simulink model "BLDCmotor_FOC_R2017b_fixdt"  (R2025a)
settings: Solver=FixedStepDiscrete  StartTime=0  StopTime=0.5  FixedStep=Ts  MaxStep=1e-6  RelTol=1e-6  AbsTol=1e-6  EnableMultiTasking=on
PreLoadFcn:
  | addpath(pwd);
  | addpath(genpath('01_Libraries'));
  | addpath(genpath('02_Figures'));
  | addpath(genpath('03_CreateParamTable'));
InitFcn:
  | init_model;
values from neighbouring files (symbols this model uses):
  a_cpr = 65535    [init_model.m]
  a_elecAngle = 60    [init_model.m]
  a_elecoffset = a_elecPeriod/12    (= 30)    [init_model.m]
  a_elecPeriod = 360    [init_model.m]
  a_fcpr = 1/65535    (= 1.52590218967e-05)    [init_model.m]
  a_mechoffset = a_elecoffset/n_polePairs    (= 5)    [init_model.m]
  a_phaAdvMax = 25    [init_model.m]
  b_angleMeasEna = 1    [init_model.m]
  b_cruiseCtrlEna = 0    [init_model.m]
  b_diagEna = 0    [init_model.m]
  b_fieldWeakEna = 0    [init_model.m]
  cf_currFilt = 0.692    [init_model.m]
  cf_idKi = Ki / (f_ctrl)    (= 0.00409061543436)    [init_model.m]
  cf_idKp = Kp    (= 0.0523598775598)    [init_model.m]
  cf_iqKi = Ki / (f_ctrl)    (= 0.00409061543436)    [init_model.m]
  cf_iqKiLimProt = 60 / (f_ctrl)    (= 0.00375)    [init_model.m]
  cf_iqKp = Kp    (= 0.0523598775598)    [init_model.m]
  cf_KbLimProt = Simulink.Parameter    [init_model.m]
  cf_nKi = 20.4 / (f_ctrl)    (= 0.001275)    [init_model.m]
  cf_nKiLimProt = 20 / (f_ctrl)    (= 0.00125)    [init_model.m]
  cf_nKp = 1.18    [init_model.m]
  cf_speedCoef = round(f_ctrl * a_mechAngle * (pi/180) * (30/pi))    [init_model.m]
  CTRL_FOC = 2    [init_model.m]
  CTRL_SIN = 1    [init_model.m]
  dV_openRate = 1000 / (f_ctrl)    (= 0.0625)    [init_model.m]
  dz_cntTrnsDetHi = 40    [init_model.m]
  dz_cntTrnsDetLo = 20    [init_model.m]
  ff_gain = ((r_motn / i_sca) * ((GD32_Vd_max_margin) / v_bus))    (= 0.338958333333)    [init_model.m]
  GD32_Vd_max_margin = GD32_Vd_max - V_margin    (= 1627)    [init_model.m]
  GD32_Vq_max_M1 = sqrt(GD32_Vd_max_margin^2 - GD32_Vq_max_XA.^2)    [init_model.m]
  i_max = i_max * i_sca    (= 500)    [init_model.m]
  id_fieldWeakMax = 5 * i_sca    (= 250)    [init_model.m]
  iq_maxSca_M1 = sqrt(1 - iq_maxSca_XA.^2)    [init_model.m]
  mcu_model = GD32F103    (= 1)    [init_model.m]
  n_commAcvLo = 15    [init_model.m]
  n_commDeacvHi = 30    [init_model.m]
  n_cruiseMotTgt = 0    [init_model.m]
  n_fieldWeakAuthHi = 300    [init_model.m]
  n_fieldWeakAuthLo = 100    [init_model.m]
  n_max = 1950    [init_model.m]
  n_polePairs = 6    [init_model.m]
  n_stdStillDet = 3    [init_model.m]
  OPEN_MODE = 0    [init_model.m]
  r_cos_M1 = cos((a_elecAngle_XA + a_elecPeriod/12)*(pi/180))    [init_model.m]
  r_errInpTgtThres = 600    [init_model.m]
  r_fieldWeakHi = 1000    [init_model.m]
  r_fieldWeakLo = 750    [init_model.m]
  r_motn = r_mot/2    (= 0.25)    [init_model.m]
  r_sin3PhaA_M1 = sin3Arm + A*r_sinPhaA_M1    [init_model.m]
  r_sin3PhaB_M1 = sin3Arm + A*r_sinPhaB_M1    [init_model.m]
  r_sin3PhaC_M1 = sin3Arm + A*r_sinPhaC_M1    [init_model.m]
  r_sin_M1 = sin((a_elecAngle_XA + a_elecPeriod/12)*(pi/180))    [init_model.m]
  SPD_MODE = 2    [init_model.m]
  STM32_Vd_max_margin = STM32_Vd_max - V_margin    (= 940)    [init_model.m]
  STM32_Vq_max_M1 = sqrt(STM32_Vd_max_margin^2 - STM32_Vq_max_XA.^2)    [init_model.m]
  t_errDequal = 1.80 * f_ctrl    (= 28800)    [init_model.m]
  t_errQual = 0.24 * f_ctrl    (= 3840)    [init_model.m]
  tgt_scale = 2047    [init_model.m]
  TRQ_MODE = 3    [init_model.m]
  Ts = 5e-6    (= 5e-06)    [init_model.m]
  Ts_ctrl = 6e-5    (= 6e-05)    [init_model.m]
  v_bus = 24    [init_model.m]
  vec_hallToPos = [0 2 0 1 4 3 5 0]    [init_model.m]
  VLT_MODE = 1    [init_model.m]
  z_commutMap_M1 = [-1 -1  0  1  1  0 ... (first row only)    [init_model.m]
  z_ctrlModReq = TRQ_MODE    (= 3)    [init_model.m]
  z_ctrlTypSel = CTRL_FOC    (= 2)    [init_model.m]
  z_maxCntRst = 2000    [init_model.m]
  z_selPhaCurMeasABC = 2    [init_model.m]
undefined symbols (not defined in the file or in its folder): BLDCmotor_FOC_R2017b_fixdt, DiscIntNeverNeededParam, DWORK0, DWORK1, DWORK2, DWORK3, powergui, spspowerguiLib
libraries: BLDC_controller_Lib x18, simulink x13, prociolib x6, eePwmGenerator x6, eePwmGeneratorMultilevel x3, mcbpositiondecoderlib x2, slpidlib x2, spsControlledVoltageSourceLib x1, spsMultimeterLib x1, spsPermanentMagnetSynchronousMachineLib x1, spsUniversalBridgeLib x1, spsVoltageMeasurementLib x1
(part 1 of 6)
Description:
  | This model implements FOC controller for a BLDC motor.
  | The controller is capable for embedded code generation.
  | 
  | Copyright © 2019-2020 Emanuel FERU
settings Model: ExtModeAutoUpdateStatusClock=off  TunableVars=Vd_max,Vq_max_M1,Vq_max_XA,a_phaAdvMax,b_angleMeasEna,b_cruiseCtrlEna,b_diagEna,b_fieldWeakEna,cf_currFilt,cf_idKi,cf_idKp,cf_iqKi,cf_iqKiLimProt,cf_iqKp,cf_nKi,cf_nKiLimProt,cf_nKp,cf_speedCoef,dV_openRate,dz_cntTrnsDetHi,dz_cntTrnsDetLo,i_max,id_fieldWeakMax,n_commAcvLo,n_commDeacvHi,n_cruiseMotTgt,n_fieldWeakAuthHi,n_fieldWeakAuthLo,n_max,n_polePairs,n_stdStillDet,r_errInpTgtThres,r_fieldWeakHi,r_fieldWeakLo,t_errDequal,t_errQual,z_ctrlTypSel,z_maxCntRst,z_selPhaCurMeasABC,sca_factor,ff_gain,a_cpr,a_fcpr  TunableVarsStorageClass=Auto,Auto,Auto,Auto,Auto,Auto,Auto,Auto,Auto,Auto,Auto,Auto,Auto,Auto,Auto,Auto,Auto,Auto,Auto,Auto,Auto,Auto,Auto,Auto,Auto,Auto,Auto,Auto,Auto,Auto,Auto,Auto,Auto,Auto,Auto,Auto,Auto,Auto,Auto,ExportedGlobal,Auto,Auto,Auto  TunableVarsTypeQualifier=,,,,,,,,,,,,,,,,,,,,,,,,,,,,,,,,,,,,,,,,,,  Creator=MathWorks  LastModifiedBy=ernes
settings SolverCC: AutoScaleAbsTol=off  AlgebraicLoopSolver=TrustRegion  AutoInsertRateTranBlk=on
settings DataIOCC: LimitDataPoints=on  SaveFormat=Array  SignalLoggingName=sigsOut
settings OptimizationCC: DefaultParameterBehavior=Inlined  UseDivisionForNetSlopeComputation=on  UseFloatMulNetSlope=on  DefaultUnderspecifiedDataType=single  UseSpecifiedMinMax=on  PassReuseOutputArgsAs=Individual arguments  ExpressionDepthLimit=2147483647.0  ZeroExternalMemoryAtStartup=off  ZeroInternalMemoryAtStartup=off  NoFixptDivByZeroProtection=on  EfficientFloat2IntCast=on  LifeSpan=1  MaxStackSize=64  SimCompilerOptimization=on  OptimizeBlockOrder=speed  DifferentSizesBufferReuse=on  EfficientTunableParamExpr=on
settings DebuggingCC: SignalRangeChecking=warning  ReadBeforeWriteMsg=DisableAll  WriteAfterWriteMsg=DisableAll  WriteAfterReadMsg=DisableAll  InheritedTsInSrcMsg=none  MultiTaskDSMMsg=none  MultiTaskCondExecSysMsg=none  ParamPrecisionLossAbsoluteDiffThreshold=10e-05  ParamPrecisionLossRelativeDiffThreshold=10e-05  ParameterTunabilityLossMsg=error  UnconnectedInputMsg=warning  UnconnectedOutputMsg=warning  UnconnectedLineMsg=warning  StateNameClashWarn=warning  SFUnexpectedBacktrackingDiag=warning  SFNoUnconditionalDefaultTransitionDiag=warning  SFExecutionAtInitializationDiag=none  ArithmeticOperatorsInVariantConditions=warning
settings HardwareCC: ProdBitPerPointer=32.0  ProdBitPerSizeT=32.0  ProdBitPerPtrDiffT=32.0  ProdLargestAtomicInteger=Long  ProdLargestAtomicFloat=Double  ProdWordSize=32.0  ProdLongLongMode=on  ProdHWDeviceType=ARM Compatible->ARM Cortex-M  TargetBitPerPointer=64.0  TargetBitPerSizeT=64.0  TargetBitPerPtrDiffT=64.0  TargetLongLongMode=on  TargetIntDivRoundTo=Zero  TargetEndianess=LittleEndian  TargetWordSize=64.0  TargetHWDeviceType=MATLAB Host  ProdEqTarget=off
settings ModelReferenceCC: UpdateModelReferenceTargets=IfOutOfDate  EnableRefExpFcnMdlSchedulingChecks=on  PropagateSignalLabelsOutOfModel=off
settings SFSimCC: SFSimEcho=off  SimUseLocalCustomCode=off  MATLABDynamicMemAlloc=off  CustomCodeUndefinedFunction=UseInterfaceOnly  SimGPUCompilerFlags="-allow-unsupported-compiler -ccbin \"C:\\Program Files (x86)\\Microsoft Visual Studio\\2022\\BuildTools\\VC\\Tools\\MSVC\\14.29.30133\\bin\\Hostx64\\x64\""
settings RTWCC: SystemTargetFile=ert.tlc  GenCodeOnly=on  TemplateMakefile=ert_default_tmf  GenerateReport=on  RetainRTWFile=on  RTWUseLocalCustomCode=off  Toolchain=GNU Tools for ARM Embedded Processors  BuildConfiguration=Faster Runs  IncludeHyperlinkInReport=on  LaunchReport=on  GenerateTraceInfo=on  GenerateTraceReport=on  GenerateTraceReportSl=on  GenerateTraceReportSf=on  GenerateTraceReportEml=on  GenerateWebview=on  GenerateCodeMetricsReport=on  GenerateCodeReplacementReport=on  GPUComputeCapability=3.5  Description=Embedded Coder
settings CodeAppCC: ForceParamTrailComments=on  IgnoreCustomStorageClasses=off  OperatorAnnotations=on  SimulinkDataObjDesc=on  SFDataObjDesc=on  CustomSymbolStrGlobalVar=rt$N$M  CustomSymbolStrType=$N$M  CustomSymbolStrFcn=$N$M$F  CustomSymbolStrMacro=$N$M  SignalNamingFcn=init_model.m  InsertBlockDesc=on
settings ERTTargetCC: ExtModeTransport=3.0  ExtModeStaticAllocSize=2048.0  InlinedParameterPlacement=Hierarchical  MultiInstanceErrorCode=None  RootIOFormat=Part of model data structure  ERTCustomFileTemplate=example_file_process.tlc  ERTFilePackagingFormat=CompactWithDataFile  PreserveStaticInFcnDecls=off  DynamicArrayContainerType=coder::array  TargetLangStandard=C99 (ISO)  IncludeMdlTerminateFcn=off  CombineSignalStateStructs=on  SuppressErrorStatus=on  CodeInterfacePackaging=Reusable function  PurelyIntegerCode=on  SupportNonFinite=off  SupportComplex=off
settings ConfigComp: CovScope=ReferencedModels  CovMetricSettings=dw  CovSaveCumulativeToWorkspaceVar=on  CovSaveSingleToWorkspaceVar=on  CovExternalEMLEnable=off  CovSFcnEnable=off
settings SimscapeCC: SimscapeNormalizeSystem=off

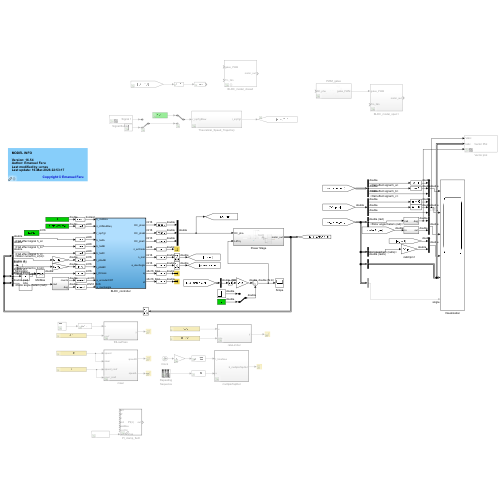
[thumbnail: Simulink's stored preview of the top-level diagram]
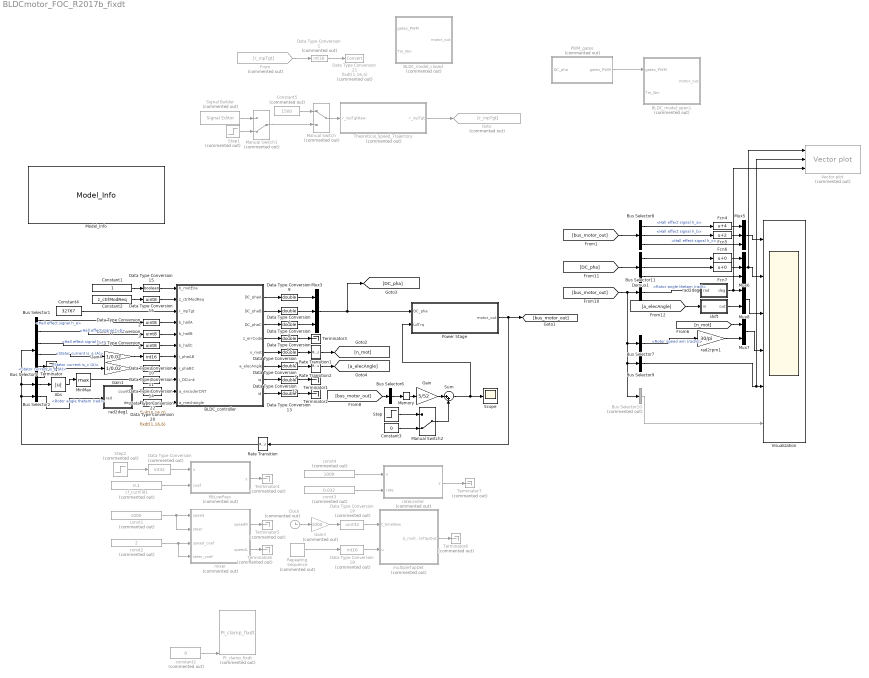
== system BLDCmotor_FOC_R2017b_fixdt ==
  Abs : Abs  SaturateOnIntegerOverflow=off
  BLDC_controller : Subsystem  TreatAsAtomicUnit=on  SystemSampleTime=Ts_ctrl
      settings: RTWFileNameOpts=Use subsystem name  FunctionWithSeparateData=on
  BLDC_model_closed : Subsystem  Commented=on
      mask help: Simulink:masks:GenSFuncDesc_MD
      mask Help: eval('feval(''rtwprivate'',''rtwhelpview'',''rtw_sfcn_block'')');
  BLDC_model_open1 : Subsystem  Commented=on
  Bus Selector1 : BusSelector  OutputSignals=Hall effect signal h_a,Hall effect signal h_b,Hall effect signal h_c,Stator current is_a (A),Stator current is_b (A),Stator current is_c (A)
  Bus Selector10 : BusSelector  Commented=on  OutputSignals=Stator back EMF e_b (V),Stator back EMF e_cV)  OutputAsBus=on
  Bus Selector11 : BusSelector  OutputSignals=Rotor angle thetam (rad)
  Bus Selector2 : BusSelector  OutputSignals=Rotor angle thetam (rad)
  Bus Selector5 : BusSelector  OutputSignals=Electromagnetic torque Te (N*m)  OutputAsBus=on
  Bus Selector6 : BusSelector  OutputSignals=Electromagnetic torque Te (N*m)  OutputAsBus=on
  Bus Selector7 : BusSelector  OutputSignals=Rotor speed wm (rad/s)
  Bus Selector8 : BusSelector  OutputSignals=Hall effect signal h_a,Hall effect signal h_b,Hall effect signal h_c
  Bus Selector9 : BusSelector  OutputSignals=Stator current is_a (A),Stator current is_b (A),Stator current is_c (A),Electromagnetic torque Te (N*m)  OutputAsBus=on
  Clock : Clock  Commented=on
  Constant1 : Constant  OutDataTypeStr=double
  Constant2 : Constant  Value=z_ctrlModReq  OutDataTypeStr=double
  Constant3 : Constant  Value=0  OutDataTypeStr=double
  Constant4 : Constant  Value=32767  OutDataTypeStr=int16
  Constant5 : Constant  Commented=on  Value=1500  OutDataTypeStr=double
  Data Type Conversion : DataTypeConversion  Commented=on  OutDataTypeStr=int32  SaturateOnIntegerOverflow=off  RndMeth=Floor
  Data Type Conversion1 : DataTypeConversion  Commented=on  OutDataTypeStr=int16  SaturateOnIntegerOverflow=off
  Data Type Conversion10 : DataTypeConversion  OutDataTypeStr=int16
  Data Type Conversion11 : DataTypeConversion  OutDataTypeStr=int16
  Data Type Conversion{5..9,12..13,17} (8 alike) : DataTypeConversion  OutDataTypeStr=double  SaturateOnIntegerOverflow=off
  Data Type Conversion14 : DataTypeConversion  OutDataTypeStr=int16
  Data Type Conversion15 : DataTypeConversion  OutDataTypeStr=boolean  SaturateOnIntegerOverflow=off
  Data Type Conversion{2..4,16} (4 alike) : DataTypeConversion  OutDataTypeStr=uint8  SaturateOnIntegerOverflow=off
  Data Type Conversion18 : DataTypeConversion  Commented=on  OutDataTypeStr=int16  SaturateOnIntegerOverflow=off  RndMeth=Floor
  Data Type Conversion19 : DataTypeConversion  Commented=on  OutDataTypeStr=uint32  SaturateOnIntegerOverflow=off  RndMeth=Floor
  Data Type Conversion20 : DataTypeConversion  OutDataTypeStr=fixdt(1,16,6)  SaturateOnIntegerOverflow=off  RndMeth=Floor
  Data Type Conversion21 : DataTypeConversion  Commented=on  OutDataTypeStr=fixdt(1,16,4)  SaturateOnIntegerOverflow=off  RndMeth=Floor
  Data Type Conversion22 : DataTypeConversion  OutDataTypeStr=fixdt(0,16,0)  SaturateOnIntegerOverflow=off  RndMeth=Floor
  Demux1 : Demux  Outputs=3
  Fcn4 : Fcn  Expr=u+4
  Fcn5 : Fcn  Expr=u+2
  Fcn6 : Fcn  Expr=u+0
  Fcn7 : Fcn  Expr=u+0
  From : From  Commented=on  GotoTag=r_inpTgt
  Gain : Gain  Gain=5/52
  Gain1 : Gain  Tag=struct('comment',struct('text','','placement',1),'logdata',struct('maxnumvals',inf,'plotchannels',[],'loggingmode',3,'channels',1),'output',struct('variable','','description','','name','$S_$B','width',1,'address','','max',NaN,'min',NaN,'class','default','type','CONTINUOUS','scaling','','lsb',1,'offset',0,'arb',0,'freeze',1,'unit','','autoscalingmode',1,'lowerheadroom',1,'upperheadroom',1,'headroomunit','bit','keepdatatype',1,'checkmin',0,'checkmax',0,'castoutput',0,'show',0),'gain',struct('variable','','description','','name','$S_$B_gain','width',1,'address','','max',NaN,'min',NaN,'class','default','type','CONTINUOUS','scaling','','lsb',1,'offset',0,'arb',0,'freeze',1,'unit','','keepdatatype',1,'value','1','scalar',0,'tolerance',1),'scalingvalid',0,'date',730486)  Gain=1/0.02  RndMeth=Zero  SaturateOnIntegerOverflow=on  OutDataTypeStr=Inherit: Same as input  ParamDataTypeStr=Inherit: Same as input
  Gain3 : Gain  Tag=struct('comment',struct('text','','placement',1),'logdata',struct('maxnumvals',inf,'plotchannels',[],'loggingmode',3,'channels',1),'output',struct('variable','','description','','name','$S_$B','width',1,'address','','max',NaN,'min',NaN,'class','default','type','CONTINUOUS','scaling','','lsb',1,'offset',0,'arb',0,'freeze',1,'unit','','autoscalingmode',1,'lowerheadroom',1,'upperheadroom',1,'headroomunit','bit','keepdatatype',1,'checkmin',0,'checkmax',0,'castoutput',0,'show',0),'gain',struct('variable','','description','','name','$S_$B_gain','width',1,'address','','max',NaN,'min',NaN,'class','default','type','CONTINUOUS','scaling','','lsb',1,'offset',0,'arb',0,'freeze',1,'unit','','keepdatatype',1,'value','1','scalar',0,'tolerance',1),'scalingvalid',0,'date',730486)  Commented=on  Gain=1000  RndMeth=Zero  SaturateOnIntegerOverflow=on  OutDataTypeStr=Inherit: Same as input  ParamDataTypeStr=Inherit: Same as input
  Gain4 : Gain  Tag=struct('comment',struct('text','','placement',1),'logdata',struct('maxnumvals',inf,'plotchannels',[],'loggingmode',3,'channels',1),'output',struct('variable','','description','','name','$S_$B','width',1,'address','','max',NaN,'min',NaN,'class','default','type','CONTINUOUS','scaling','','lsb',1,'offset',0,'arb',0,'freeze',1,'unit','','autoscalingmode',1,'lowerheadroom',1,'upperheadroom',1,'headroomunit','bit','keepdatatype',1,'checkmin',0,'checkmax',0,'castoutput',0,'show',0),'gain',struct('variable','','description','','name','$S_$B_gain','width',1,'address','','max',NaN,'min',NaN,'class','default','type','CONTINUOUS','scaling','','lsb',1,'offset',0,'arb',0,'freeze',1,'unit','','keepdatatype',1,'value','1','scalar',0,'tolerance',1),'scalingvalid',0,'date',730486)  Gain=1/0.02  RndMeth=Zero  SaturateOnIntegerOverflow=on  OutDataTypeStr=Inherit: Same as input  ParamDataTypeStr=Inherit: Same as input
  Goto : Goto  Commented=on  GotoTag=r_inpTgt
  Manual Switch : ManualSwitch  Commented=on
  Manual Switch1 : ManualSwitch  Commented=on  CurrentSetting=0
  Manual Switch2 : ManualSwitch  CurrentSetting=0
  Memory : Memory
  MinMax : MinMax  Function=max
  Model_Info : BLDC_controller_Lib/Model_Info
  Mux3 : Mux  Inputs=3
  Mux5 : Mux  Inputs=3
  Mux6 : Mux  Inputs=3
  Mux7 : Mux  Inputs=2
  Mux8 : Mux  Inputs=2
  PI_clamp_fixdt : BLDC_controller_Lib/PI_clamp_fixdt  Commented=on  SystemSampleTime=-1  VariantActivationTime=update diagram  EmptyChoice=off  PassThrough=off  PassThroughVariantControl=(default)  EmptyChoiceVariantControl=(default)  AllowFlexibleInterface=on  Latency=0  AutoFrameSizeCalculation=off
  PWM_gates : Subsystem  Commented=on
  Power Stage : Subsystem
  Rate Transition : RateTransition  Integrity=off  Deterministic=off
  Rate Transition1 : RateTransition  Integrity=off  Deterministic=off
  Rate Transition2 : RateTransition
  Repeating Sequence : simulink/Sources/Repeating Sequence  Commented=on  rep_seq_t=[0 0.4 0.8 1.2 1.6 3]  rep_seq_y="[0 900  0  900 0 0]"
  Scope : Scope
      settings: ActiveDisplayYMinimum=-7.8527501814410146  ActiveDisplayYMaximum=12.467804815111347  DataLoggingVariableName=ScopeData2
  Signal Builder : SignalEditorBlockLib/Signal Editor  Commented=on  FileName=SignalBuilder_2.mat  ActiveScenario=Group_1  ActiveSignal=Signal 1  IsBus=off  OutputBusObjectStr=Bus: BusObject  SampleTime=-1  OutputAfterFinalValue=Extrapolation  Unit=inherit  PreserveSignalName=on  ApplySigPropsToAllScenarios=on  ApplySigPropsToAllSignals=off  SignalPropertySource=Dialog parameters
  Step : Step  Time=0.25  Before=-5  After=5  SampleTime=0
  Step1 : Step  Commented=on  Time=0.25  Before=1500  After=-1500
  Step2 : Step  Commented=on  Time=0.25  Before=20000  After=0  OutDataTypeStr=single  SampleTime=0
  Sum : Sum  Inputs=|++
  Terminator{,1..3} (4 alike) : Terminator
      Terminator1 settings: Tag=Controls_Lib  Description=Terminator  CopyFcn=Lib_CopyFcn(gcb);  PreDeleteFcn=Lib_PreDeleteFcn(gcb);
      Terminator2 settings: Tag=Controls_Lib  Description=Terminator  CopyFcn=Lib_CopyFcn(gcb);  PreDeleteFcn=Lib_PreDeleteFcn(gcb);
      Terminator3 settings: Tag=Controls_Lib  Description=Terminator  CopyFcn=Lib_CopyFcn(gcb);  PreDeleteFcn=Lib_PreDeleteFcn(gcb);
  Terminator{4..8} (5 alike) : Terminator  Commented=on
      settings: Tag=Controls_Lib  Description=Terminator  CopyFcn=Lib_CopyFcn(gcb);  PreDeleteFcn=Lib_PreDeleteFcn(gcb);
  Theoretical_Speed_Trajectory : Subsystem  Commented=on
  Vector plot : mcbutilslib/Vector plot  Commented=on  InputSignals=Vabc Iabc Theta  ReferenceFrame=Rotating Reference Frame  axisAlign=Q-axis  thetaUnits=Degrees  angleUnits=Radians  OpenFigAtSimStart=off  debugEnable=0
      settings: LibrarySourceBlock=mcblib/Signal Management/Vector plot
  Visualization : Scope  NumInputPorts=6
      settings: TimeSpan=0.2  ActiveDisplayString=4  ActiveDisplayYMinimum=-21.20436412488284  ActiveDisplayYMaximum=402.88291837277404
  cf_currFilt1 : Constant  Commented=on  Value=0.1  OutDataTypeStr=fixdt(0,16,16)
  const1 : Constant  Commented=on  Value=1000  OutDataTypeStr=fixdt(1,16,4)
  const2 : Constant  Commented=on  Value=2  OutDataTypeStr=fixdt(1,16,14)
  const3 : Constant  Commented=on  Value=0.032  OutDataTypeStr=fixdt(1,16,4)
  const4 : Constant  Commented=on  Value=1000  OutDataTypeStr=int16
  constant2 : Constant  Commented=on  Value=0  OutDataTypeStr=Inherit: Inherit via back propagation
  filtLowPass : Subsystem  Commented=on  TreatAsAtomicUnit=on  SystemSampleTime=Ts_ctrl
      settings: RTWFcnNameOpts=Use subsystem name
  mixer : Subsystem  Commented=on  TreatAsAtomicUnit=on  SystemSampleTime=Ts_ctrl
      settings: RTWFcnNameOpts=Use subsystem name
  multipleTapDet : Subsystem  Commented=on  TreatAsAtomicUnit=on
      settings: RTWFcnNameOpts=Use subsystem name
  rad2deg : Subsystem
  rad2deg1 : Subsystem
  rad2rpm1 : Gain  Gain=30/pi
  rateLimiter : Subsystem  Commented=on  TreatAsAtomicUnit=on  SystemSampleTime=Ts_ctrl
      settings: RTWFcnNameOpts=Use subsystem name
  shift : Subsystem
  wires:
  BLDC_controller/5(n_mot) -> Data Type Conversion7/1
  Sum/1 -> Scope/1, Power Stage/2(LdTrq)
  Bus Selector1/2 -> Data Type Conversion3/1  "<Hall effect signal h_b>"
  Bus Selector1/1 -> Data Type Conversion2/1  "<Hall effect signal h_a>"
  Bus Selector1/3 -> Data Type Conversion4/1  "<Hall effect signal h_c>"
  Data Type Conversion2/1 -> BLDC_controller/4("b_hallA ")
  Data Type Conversion3/1 -> BLDC_controller/5(b_hallB)
  Data Type Conversion4/1 -> BLDC_controller/6(b_hallC)
  BLDC_controller/2(DC_phaB) -> Data Type Conversion6/1
  BLDC_controller/3(DC_phaC) -> Data Type Conversion8/1
  BLDC_controller/1(DC_phaA) -> Data Type Conversion9/1
  Data Type Conversion7/1 -> Rate Transition1/1
  BLDC_controller/6(a_elecAngle) -> Data Type Conversion5/1
  Mux3/1 -> Power Stage/1(DC_pha), [DC_pha]
  Rate Transition1/1 -> [n_mot]
  Manual Switch/1 -> Theoretical_Speed_Trajectory/1(r_inpTgtRaw)
  Constant5/1 -> Manual Switch/1
  Signal Builder/1 -> Manual Switch1/1
  Manual Switch1/1 -> Manual Switch/2
  Step1/1 -> Manual Switch1/2
  Data Type Conversion8/1 -> Mux3/3
  Data Type Conversion6/1 -> Mux3/2
  Data Type Conversion9/1 -> Mux3/1
  Data Type Conversion10/1 -> BLDC_controller/7(i_phaAB)
  Data Type Conversion11/1 -> BLDC_controller/8(i_phaBC)
  Gain4/1 -> Data Type Conversion10/1
  Gain1/1 -> Data Type Conversion11/1
  BLDC_controller/7(iq) -> Data Type Conversion12/1
  Data Type Conversion13/1 -> Terminator2/1
  BLDC_controller/8(id) -> Data Type Conversion13/1
  MinMax/1 -> Data Type Conversion14/1
  Data Type Conversion14/1 -> BLDC_controller/9(i_DCLink)
  Bus Selector1/4 -> Gain4/1  "<Stator current is_a (A)>"
  Data Type Conversion15/1 -> BLDC_controller/1(b_motEna)
  Constant1/1 -> Data Type Conversion15/1
  [bus_motor_out] -> Bus Selector6/1
  Bus Selector6/1 -> Memory/1
  Gain/1 -> Sum/1
  Data Type Conversion16/1 -> BLDC_controller/2(z_ctrlModReq)
  Constant2/1 -> Data Type Conversion16/1
  Rate Transition/1 -> Bus Selector2/1, Bus Selector1/1, Bus Selector5/1
  Memory/1 -> Gain/1
  Step/1 -> Manual Switch2/1
  Manual Switch2/1 -> Sum/2
  Constant3/1 -> Manual Switch2/2
  Data Type Conversion17/1 -> Terminator3/1
  BLDC_controller/4(z_errCode) -> Data Type Conversion17/1
  Data Type Conversion12/1 -> Terminator1/1
  Bus Selector5/1 -> Abs/1
  Abs/1 -> MinMax/1
  filtLowPass/1(y) -> Terminator4/1
  cf_currFilt1/1 -> filtLowPass/2(coef)
  Data Type Conversion/1 -> filtLowPass/1(u)
  mixer/1(speedR) -> Terminator5/1
  const1/1 -> mixer/2(steer), mixer/1(speed)
  const2/1 -> mixer/4(steer_coef), mixer/3(speed_coef)
  mixer/2(speedL) -> Terminator6/1
  Gain3/1 -> Data Type Conversion19/1
  Data Type Conversion19/1 -> multipleTapDet/1(t_timeNow)
  Data Type Conversion18/1 -> multipleTapDet/2(u)
  multipleTapDet/1(b_multipleTapOut) -> Terminator8/1
  Repeating Sequence/1 -> Data Type Conversion18/1
  Clock/1 -> Gain3/1
  Bus Selector8/1 -> Fcn4/1  "<Hall effect signal h_a>"
  [a_elecAngle] -> shift/1(in)
  rad2deg/1(deg) -> Vector plot/3, Mux8/1
  Mux8/1 -> Visualization/3
  [DC_pha] -> Demux1/1
  rad2rpm1/1 -> Mux7/2
  Fcn6/1 -> Mux6/1
  Bus Selector8/2 -> Fcn5/1  "<Hall effect signal h_b>"
  Mux7/1 -> Visualization/4
  Demux1/3 -> Mux6/3
  Fcn7/1 -> Mux6/2
  Mux6/1 -> Visualization/2, Vector plot/1
  Demux1/2 -> Fcn7/1
  Demux1/1 -> Fcn6/1
  Bus Selector10/1 -> Visualization/6
  [bus_motor_out] -> Bus Selector11/1, Bus Selector9/1, Bus Selector10/1, Bus Selector7/1
  [n_mot] -> Mux7/1
  Bus Selector7/1 -> rad2rpm1/1  "<Rotor speed wm (rad/s)>"
  Bus Selector9/1 -> Vector plot/2, Visualization/5
  Rate Transition2/1 -> [a_elecAngle]
  Data Type Conversion5/1 -> Rate Transition2/1
  shift/1(out) -> Mux8/2
  Bus Selector2/1 -> rad2deg1/1(rad)  "<Rotor angle thetam (rad)>"
  Bus Selector11/1 -> rad2deg/1(rad)  "<Rotor angle thetam (rad)>"
  Constant4/1 -> BLDC_controller/3(r_inpTgt)
  rad2deg1/2(deg) -> Data Type Conversion20/1
  const3/1 -> rateLimiter/2(rate)
  Step2/1 -> Data Type Conversion/1
  rateLimiter/1(y) -> Terminator7/1
  const4/1 -> rateLimiter/1(u)
  Theoretical_Speed_Trajectory/1(r_inpTgt) -> Goto/1
  constant2/1 -> PI_clamp_fixdt/7
  From/1 -> Data Type Conversion1/1
  Data Type Conversion1/1 -> Data Type Conversion21/1
  Bus Selector1/6 -> Gain1/1  "<Stator current is_c (A)>"
  Bus Selector1/5 -> Terminator/1  "<Stator current is_b (A)>"
  Data Type Conversion20/1 -> BLDC_controller/11(a_mechangle)
  rad2deg1/1(counts) -> Data Type Conversion22/1
  Data Type Conversion22/1 -> BLDC_controller/10(a_encoderCNT)
  Power Stage/1(motor_out) -> Rate Transition/1, [bus_motor_out]
  [bus_motor_out] -> Bus Selector8/1
  Bus Selector8/3 -> Mux5/3  "<Hall effect signal h_c>"
  Fcn4/1 -> Mux5/1
  Fcn5/1 -> Mux5/2
  Mux5/1 -> Visualization/1
  PWM_gates/1(gates_PWM) -> BLDC_model_open1/1(gates_PWM)

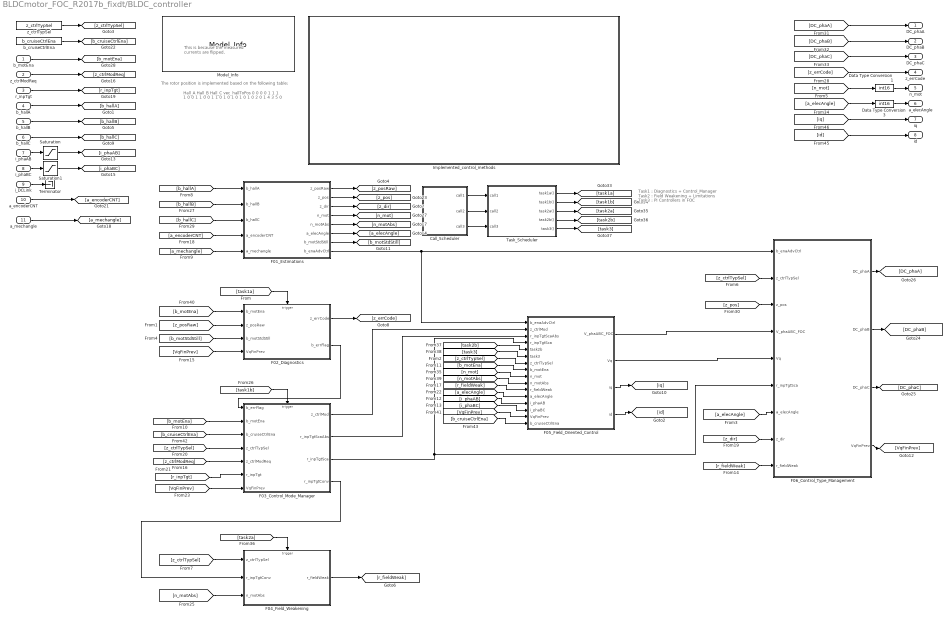
== system BLDCmotor_FOC_R2017b_fixdt/BLDC_controller ==
  note: Task1 : Diagnostics + Control_Manager
      |
      | Task2 : Field Weakening + Limitations
      |
      | Task3 : PI Controllers in FOC
  note: The rotor position is implemented based on the following table:
  note: Hall_A
      | Hall_B
      | Hall_C
      | vec_hallToPos
      |
      | 0
      | 0
      | 0
      | 0
      | 1
      | 1
      | 1
      | 1
      | 0
      | 0
      | 1
      | 1
      | 0
      | 0
      | 1
      | 1
      | 0
      | 1
      | 0
      | 1
      | 0
      | 1
      | 0
      | 1
      | 0
      | 2
      | 0
      | 1
      | 4
      | 3
      | 5
      | 0
  note: This is because the measured currents are flipped.
  b_motEna : Inport
  z_ctrlModReq : Inport  Port=2
  r_inpTgt : Inport  Port=3
  "b_hallA " : Inport  Port=4
  b_hallB : Inport  Port=5
  b_hallC : Inport  Port=6
  i_phaAB : Inport  Port=7
  i_phaBC : Inport  Port=8
  i_DCLink : Inport  Port=9
  a_encoderCNT : Inport  Port=10
  a_mechangle : Inport  Port=11
  Call_Scheduler : Subsystem
  Data Type Conversion1 : DataTypeConversion  OutDataTypeStr=int16  SaturateOnIntegerOverflow=off  RndMeth=Floor
  Data Type Conversion3 : DataTypeConversion  OutDataTypeStr=int16  SaturateOnIntegerOverflow=off  RndMeth=Floor
  F01_Estimations : Subsystem
  F02_Diagnostics : Subsystem
  F03_Control_Mode_Manager : Subsystem
  F04_Field_Weakening : Subsystem
  F05_Field_Oriented_Control : Subsystem
  F06_Control_Type_Management : Subsystem
  Implemented_control_methods : Subsystem
      mask Display: image('control_methods.png')
  Model_Info : BLDC_controller_Lib/Model_Info
  Saturation : Saturate  UpperLimit=1700  LowerLimit=-1700  OutDataTypeStr=fixdt(1,16,4)
  Saturation1 : Saturate  UpperLimit=1700  LowerLimit=-1700  OutDataTypeStr=fixdt(1,16,4)
  Task_Scheduler : Stateflow chart  TreatAsAtomicUnit=on
  Terminator : Terminator
  b_cruiseCtrlEna : Constant  Value=b_cruiseCtrlEna  OutDataTypeStr=boolean
  z_ctrlTypSel : Constant  Value=z_ctrlTypSel  OutDataTypeStr=uint8
  DC_phaA : Outport  VectorParamsAs1DForOutWhenUnconnected=off
  DC_phaB : Outport  Port=2  VectorParamsAs1DForOutWhenUnconnected=off
  DC_phaC : Outport  Port=3  VectorParamsAs1DForOutWhenUnconnected=off
  z_errCode : Outport  Port=4  OutputWhenDisabled=reset  InitialOutput=0  VectorParamsAs1DForOutWhenUnconnected=off
  n_mot : Outport  Port=5  VectorParamsAs1DForOutWhenUnconnected=off
  a_elecAngle : Outport  Port=6  VectorParamsAs1DForOutWhenUnconnected=off
  iq : Outport  Port=7  OutputWhenDisabled=reset  InitialOutput=0  VectorParamsAs1DForOutWhenUnconnected=off
  id : Outport  Port=8  OutputWhenDisabled=reset  InitialOutput=0  VectorParamsAs1DForOutWhenUnconnected=off
  wires:
  [n_mot] -> F05_Field_Oriented_Control/9(n_mot)
  F02_Diagnostics/2(b_errFlag) -> F03_Control_Mode_Manager/1(b_errFlag)
  [id] -> id/1
  [iq] -> iq/1
  i_phaBC/1 -> Saturation1/1
  [z_pos] -> F06_Control_Type_Management/3(z_pos)
  Saturation/1 -> [i_phaAB]
  F01_Estimations/5(n_motAbs) -> [n_motAbs]
  [z_errCode] -> z_errCode/1
  [r_fieldWeak] -> F05_Field_Oriented_Control/11(r_fieldWeak)
  [DC_phaB] -> DC_phaB/1
  [z_ctrlTypSel] -> F06_Control_Type_Management/2(z_ctrlTypSel)
  [z_posRaw] -> F02_Diagnostics/2(z_posRaw)
  Data Type Conversion1/1 -> n_mot/1
  [i_phaAB] -> F05_Field_Oriented_Control/13(i_phaAB)
  i_phaAB/1 -> Saturation/1
  F05_Field_Oriented_Control/1(V_phaABC_FOC) -> F06_Control_Type_Management/4(V_phaABC_FOC)
  [i_phaBC] -> F05_Field_Oriented_Control/14(i_phaBC)
  [n_mot] -> Data Type Conversion1/1
  [DC_phaC] -> DC_phaC/1
  F06_Control_Type_Management/2(DC_phaB) -> [DC_phaB]
  z_ctrlModReq/1 -> [z_ctrlModReq]
  F06_Control_Type_Management/1(DC_phaA) -> [DC_phaA]
  F01_Estimations/4("n_mot ") -> [n_mot]
  F05_Field_Oriented_Control/4(id) -> [id]
  F01_Estimations/6(a_elecAngle) -> [a_elecAngle]
  [b_hallB] -> F01_Estimations/2(b_hallB)
  i_DCLink/1 -> Terminator/1
  F05_Field_Oriented_Control/3(iq) -> [iq]
  [a_elecAngle] -> Data Type Conversion3/1
  F06_Control_Type_Management/3("DC_phaC ") -> [DC_phaC]
  Saturation1/1 -> [i_phaBC]
  b_hallB/1 -> [b_hallB]
  F01_Estimations/8(b_enaAdvCtrl) -> F05_Field_Oriented_Control/1(b_enaAdvCtrl), F06_Control_Type_Management/1(b_enaAdvCtrl)
  F02_Diagnostics/1("z_errCode ") -> [z_errCode]
  b_motEna/1 -> [b_motEna]
  b_hallC/1 -> [b_hallC]
  [a_elecAngle] -> F05_Field_Oriented_Control/12(a_elecAngle)
  [DC_phaA] -> DC_phaA/1
  F01_Estimations/1(z_posRaw) -> [z_posRaw]
  F03_Control_Mode_Manager/1(z_ctrlMod) -> F05_Field_Oriented_Control/2(z_ctrlMod)
  [b_hallA] -> F01_Estimations/1(b_hallA)
  "b_hallA "/1 -> [b_hallA]
  F01_Estimations/2(z_pos) -> [z_pos]
  z_ctrlTypSel/1 -> [z_ctrlTypSel]
  [b_hallC] -> F01_Estimations/3(b_hallC)
  [b_motStdStill] -> F02_Diagnostics/3(b_motStdStill)
  F01_Estimations/7(b_motStdStill) -> [b_motStdStill]
  [VqFinPrev] -> F02_Diagnostics/4(VqFinPrev)
  F06_Control_Type_Management/4(VqFinPrev) -> [VqFinPrev]
  [b_motEna] -> F05_Field_Oriented_Control/8(b_motEna)
  F03_Control_Mode_Manager/3(r_inpTgtSca) -> F05_Field_Oriented_Control/4(r_inpTgtSca), F06_Control_Type_Management/6(r_inpTgtSca)
  F05_Field_Oriented_Control/2(Vq) -> F06_Control_Type_Management/5(Vq)
  [a_elecAngle] -> F06_Control_Type_Management/7(a_elecAngle)
  [r_fieldWeak] -> F06_Control_Type_Management/9(r_fieldWeak)
  F01_Estimations/3(z_dir) -> [z_dir]
  [z_dir] -> F06_Control_Type_Management/8(z_dir)
  F04_Field_Weakening/1("r_fieldWeak ") -> [r_fieldWeak]
  [n_motAbs] -> F04_Field_Weakening/3(n_motAbs)
  [task3] -> F05_Field_Oriented_Control/6(task3)
  [task2b] -> F05_Field_Oriented_Control/5(task2b)
  [n_motAbs] -> F05_Field_Oriented_Control/10(n_motAbs)
  [b_motEna] -> F02_Diagnostics/1(b_motEna)
  [b_motEna] -> F03_Control_Mode_Manager/2(b_motEna)
  [z_ctrlTypSel] -> F03_Control_Mode_Manager/4(z_ctrlTypSel)
  [z_ctrlModReq] -> F03_Control_Mode_Manager/5(z_ctrlModReq)
  [VqFinPrev] -> F03_Control_Mode_Manager/7(VqFinPrev)
  [r_inpTgt] -> F03_Control_Mode_Manager/6(r_inpTgt)
  a_encoderCNT/1 -> [a_encoderCNT]
  [a_encoderCNT] -> F01_Estimations/4(a_encoderCNT)
  [VqFinPrev] -> F05_Field_Oriented_Control/15(VqFinPrev)
  [b_cruiseCtrlEna] -> F03_Control_Mode_Manager/3(b_cruiseCtrlEna)
  [b_cruiseCtrlEna] -> F05_Field_Oriented_Control/16(b_cruiseCtrlEna)
  b_cruiseCtrlEna/1 -> [b_cruiseCtrlEna]
  Data Type Conversion3/1 -> a_elecAngle/1
  [task1b] -> F03_Control_Mode_Manager/Trigger
  [task2a] -> F04_Field_Weakening/Trigger
  [task1a] -> F02_Diagnostics/Trigger
  F03_Control_Mode_Manager/2(r_inpTgtScaAbs) -> F05_Field_Oriented_Control/3(r_inpTgtScaAbs)
  Task_Scheduler/4(task2b()) -> [task2b]
  Task_Scheduler/3(task2a()) -> [task2a]
  Task_Scheduler/2(task1b()) -> [task1b]
  Task_Scheduler/1(task1a()) -> [task1a]
  Task_Scheduler/5(task3()) -> [task3]
  Call_Scheduler/2(call2) -> Task_Scheduler/2(call2)
  Call_Scheduler/1(call1) -> Task_Scheduler/1(call1)
  Call_Scheduler/3(call3) -> Task_Scheduler/3(call3)
  [z_ctrlTypSel] -> F05_Field_Oriented_Control/7(z_ctrlTypSel)
  [z_ctrlTypSel] -> F04_Field_Weakening/1(z_ctrlTypSel)
  a_mechangle/1 -> [a_mechangle]
  [a_mechangle] -> F01_Estimations/5(a_mechangle)
  F03_Control_Mode_Manager/4(r_inpTgtConv) -> F04_Field_Weakening/2(r_inpTgtConv)
  r_inpTgt/1 -> [r_inpTgt]

== system BLDCmotor_FOC_R2017b_fixdt/BLDC_model_closed ==
  gates_PWM : Inport
  Tm_Nm : Inport  Port=2
  BLDC_model_sfcn : S-Function  FunctionName=BLDC_model_sf  SFunctionModules=""  SFunctionDeploymentMode=off  EnableBusSupport=off  SFcnStateName=DWORK0,DWORK1,DWORK2,DWORK3  mask{rtw_sf_name=BLDC_model_sf, showVar=off}
      mask prompts: rtw_sf_name "Simulink:masks:GenSFuncName_MP"; showVar "Simulink:masks:GenSFuncShowModuleList_MP"
      mask help: Simulink:masks:GenSFuncDesc_MD
      mask init:
      | displist = '';
      | if ~strcmp(get_param(gcb, 'FunctionName'), rtw_sf_name);
      |   set_param(gcb, 'FunctionName', rtw_sf_name);
      | end
      | % Check if we are generating code
      | rtw_mode = false;
      | if strcmpi(get_param(bdroot(gcb),'SimulationStatus'),'Initializing')
      | 	rtw_mode = strcmpi(get_param(bdroot(gcb),'BuildingRTWCode'),'on') && ...
      | 		~strcmpi(get_param(bdroot(gcb),'TargetStyle'),'SimulationTarget');
      | end
      | if showVar || rtw_mode
      | 	if exist('rtwsfunc') == 2 | exist('rtwsfunc') == 6
      | 		tmplist = rtwsfunc(rtw_sf_name,gcb);
      | 		tmplist = DAStudio.message('Simulink:masks:GenSFuncListOfModules_IC', tmplist);
      | 	elseif showVar
      | 		tmplist1 = DAStudio.message('Simulink:masks:GenSFuncListOfModules_IC', '');
      |         tmplist2 = DAStudio.message('Simulink:masks:GenSFuncNotLicensed_IC');
      |         tmplist = [tmplist1 tmplist2];
      |  	end
      | end
      | if showVar
      |   displist = tmplist;
      | end
      settings: SFcnIsStateOwnerBlock=on
      settings: CopyFcn=|
      | if ~strcmp(get_param(gcb,'Linkstatus'),'none') && ...
      | ~strcmp(get_param(gcb,'Linkstatus'),'implicit')
      |   set_param(gcb,'LinkStatus','none');
      | end
      mask Help: eval('feval(''rtwprivate'',''rtwhelpview'',''rtw_sfcn_block'')');
      mask Display:
      | port_label('input',1,'gates_PWM');
      | port_label('input',2,'Tm_Nm');
      | port_label('output',1,'Stator current is_a (A)');
      | port_label('output',2,'Stator current is_b (A)');
      | port_label('output',3,'Stator current is_c (A)');
      | port_label('output',4,'Stator back EMF e_a (V)');
      | port_label('output',5,'Stator back EMF e_b (V)');
      | port_label('output',6,'Stator back EMF e_cV)');
      | port_label('output',7,'Hall effect signal h_a');
      | port_label('output',8,'Hall effect signal h_b');
      | port_label('output',9,'Hall effect signal h_c');
      | port_label('output',10,'Rotor speed wm (rad/s)');
      | port_label('output',11,'Rotor angle thetam (rad)');
      | port_label('output',12,'Electromagnetic torque Te (N*m)');
  __InputSSForSFun__ : Subsystem
  __OutputSSForSFun__ : Subsystem
  motor_out : Outport  VectorParamsAs1DForOutWhenUnconnected=off
  wires:
  gates_PWM/1 -> __InputSSForSFun__/1(gates_PWM)
  Tm_Nm/1 -> __InputSSForSFun__/2(Tm_Nm)
  __InputSSForSFun__/1(__UniqueOutportName__1__) -> BLDC_model_sfcn/1
  __InputSSForSFun__/2(__UniqueOutportName__2__) -> BLDC_model_sfcn/2
  BLDC_model_sfcn/1 -> __OutputSSForSFun__/1(__UniqueInportName__1__)
  BLDC_model_sfcn/2 -> __OutputSSForSFun__/2(__UniqueInportName__2__)
  BLDC_model_sfcn/3 -> __OutputSSForSFun__/3(__UniqueInportName__3__)
  BLDC_model_sfcn/4 -> __OutputSSForSFun__/4(__UniqueInportName__4__)
  BLDC_model_sfcn/5 -> __OutputSSForSFun__/5(__UniqueInportName__5__)
  BLDC_model_sfcn/6 -> __OutputSSForSFun__/6(__UniqueInportName__6__)
  BLDC_model_sfcn/7 -> __OutputSSForSFun__/7(__UniqueInportName__7__)
  BLDC_model_sfcn/8 -> __OutputSSForSFun__/8(__UniqueInportName__8__)
  BLDC_model_sfcn/9 -> __OutputSSForSFun__/9(__UniqueInportName__9__)
  BLDC_model_sfcn/10 -> __OutputSSForSFun__/10(__UniqueInportName__10__)
  BLDC_model_sfcn/11 -> __OutputSSForSFun__/11(__UniqueInportName__11__)
  BLDC_model_sfcn/12 -> __OutputSSForSFun__/12(__UniqueInportName__12__)
  __OutputSSForSFun__/1(motor_out) -> motor_out/1

== system BLDCmotor_FOC_R2017b_fixdt/BLDC_model_open1 ==
  gates_PWM : Inport
  Tm_Nm : Inport  Port=2
  Constant1 : Constant  Value=v_bus
  Controlled Voltage Source1 : spsControlledVoltageSourceLib/Controlled Voltage Source  Initialize=on  Source_Type=DC  Amplitude=v_bus  Phase=0  Frequency=0  Measurements=Voltage
  Multimeter : spsMultimeterLib/Multimeter  L=17  sel=[1 2 3 4 5 6 7 8 9 10 11 12 13 14 15 16 17]  yselected={}  Gain=[1 1 1 1 1 1 1 1 1 1 1 1 1 1 1 1 1]  OutputType=Complex  PlotAtSimulationStop=off  PhasorSimulation=off
  Permanent Magnet Synchronous Machine : spsPermanentMagnetSynchronousMachineLib/Permanent Magnet Synchronous Machine  NbPhases=3  FluxDistribution=Sinusoidal  RotorType=Round  MechanicalLoad=Torque Tm  PresetModel=No  ShowDetailedParameters=on  MeasurementBus=off  Resistance=r_motn  Inductance=0.0002  dqInductances=[8.5e-3, 8.5e-3]  La=0.0005  MachineConstant=Torque Constant (N.m / A_peak)  Flux=0.11111  VoltageCst=120.92  TorqueCst=1  Flat=120  Mechanical=[10 0.1 n_polePairs 0.01]  PolePairs=n_polePairs  InitialConditions=[0,0, 0,0]  InitialConditions5ph=[0 0 0 0 0 0]  RefAngle=Aligned with phase A axis (original Park)  IterativeDiscreteModel=Trapezoidal non iterative  TsBlock=-1  TsPowergui=0
  Scope : Scope
      settings: ActiveDisplayYMinimum=1.1443899942205835  ActiveDisplayYMaximum=24.171247204109754  DataLoggingVariableName=ScopeData10
  Universal Bridge : spsUniversalBridgeLib/Universal Bridge  Arms=3  SnubberResistance=5000  SnubberCapacitance=inf  Device=MOSFET / Diodes  Ron=1e-4  Lon=0  ForwardVoltages="[  0  0  ]"  ForwardVoltage=0  GTOparameters=[ 10e-6 , 20e-6 ]  IGBTparameters=[ 1e-6 , 2e-6 ]  Measurements=All voltages and currents  Measurements_2=None  converterType=Rectifier
  Vdc : Scope
      settings: TimeSpan=0.2  Title=DC bus voltage  ActiveDisplayYMinimum=3.1740568090426393  ActiveDisplayYMaximum=81.954012559433338  DataLoggingVariableName=ScopeData2  DataLoggingSaveFormat=Structure
  Voltage Measurement1 : spsVoltageMeasurementLib/Voltage Measurement  PhasorSimulation=off  OutputType=Complex  PSBequivalent=0
  powergui : Subsystem  Priority=2  AncestorBlock=spspowerguiLib/powergui  InitFcn=powergui( 'InitFcn_Callback' , gcb , 0 , [ ] );  mask(PSB option menu block){SimulationMode=Discrete, SampleTime=Ts, frequency=60, Iterations=50, frequencyindice=0, Pbase=100e6, ErrMax=1e-4, UnitsV=kV, UnitsW=MW, buscounter=0, FunctionMessages=off, echomessages=off, EnableUseOfTLC=off, CurrentSourceSwitches=off, DisableSnubberDevices=off, DisableRonSwitches=off, DisableVfSwitches=off, DisplayEquations=off, AutomaticDiscreteSolvers=off, SolverType=Tustin/Backward Euler (TBE), Interpol=off, ExternalGateDelay=off, methode=off, Ts=0, x0status=blocks, SPID=off, SwTol=0, HookPort=off, NonlinearTolerance=1e-4, nMaxIteration=100, ContinueOnMaxIteration=off, RestoreLinks=warning, ResistiveCurrentMeasurement=off, Frange=[0:2:500], Ylog=off, Xlog=on, ShowGrid=off, save=off, variable=ZData, structure=0, ZoomFFT=on, StartTime=0.0, cycles=1, DisplayStyle=1, fundamental=60, FreqAxis=off, MaxFrequency=1000, frequencyindicesteady=1, RmsSteady=1, display=off}
      mask prompts: SimulationMode "Simulation type:"; SampleTime "Sample time (s):"; frequency "Frequency (Hz):"; Iterations "Max iterations"; frequencyindice "Frequency (Hz)"; Pbase "Base power (VA)"; ErrMax "PQ tolerance (pu)"; UnitsV "Voltage units"; UnitsW "Power units"; buscounter "Load flow bus counter"; FunctionMessages "Disable Specialized Power Systems warnings"; echomessages "Display Specialized Power Systems compilation messages"; EnableUseOfTLC "Use TLC file when in Accelerator Simulation Mode and for code generation"; CurrentSourceSwitches "Disable ideal switching"; DisableSnubberDevices "Disable snubbers in switching devices"; DisableRonSwitches "Disable Ron resistances in switching devices"; DisableVfSwitches "Disable forward voltages in switching devices"; DisplayEquations "Display circuit differential equations"; AutomaticDiscreteSolvers "Automatically handle Discrete solver and Advanced tab solver settings of blocks"; SolverType "Discrete solver"; Interpol "Interpolate switching events"; ExternalGateDelay "Use time-stamped gate signals"; methode "Store switching topologies"; Ts "Buffer size (MBytes):"; x0status "Start simulation with initial electrical states from:"; SPID "Use ideal switching devices"; SwTol "Switch tolerance"; HookPort "Allow multiple powergui blocks"; NonlinearTolerance "Solver tolerance"; nMaxIteration "Maximum number of iterations"; ContinueOnMaxIteration "Continue Simulation if maximum number of iterations is reached"; RestoreLinks "Restore disabled links of Simscape Power Systems ST blocks:"; ResistiveCurrentMeasurement "Use non ideal current measurement blocks (1e-4Ohm internal resistance)"; Frange "Frequency Range"; Ylog "Log impedance"; Xlog "log Frequency"; ShowGrid "grid"; save "Save Data To Workspace"; variable "Variable Name"; structure "Structure Name (PSBFFTSCOPE)"; ZoomFFT "ZoomFFT (PSBFFTSCOPE)"; StartTime "Start Time (PSBFFTSCOPE)"; cycles "Cycles (PSBFFTSCOPE)"; DisplayStyle "Display style (PSBFFTSCOPE)"; fundamental "Fundamental (PSBFFTSCOPE)"; FreqAxis "Frequency Axis (PSBFFTSCOPE)"; MaxFrequency "Max Frequency (PSBFFTSCOPE)"; frequencyindicesteady "Frequency indice (STEADYSTATE)"; RmsSteady "RMS display (STEADYSTATE)"; display "Display Results"
      mask help: Set simulation type, simulation parameters, and preferences.
      mask init:
      | dispMessage = '';
      | dispMessage = powergui('MaskInitialization',gcb,SimulationMode,SampleTime);
      settings: PreSaveFcn=powergui( 'PreSaveFcn_Callback' , gcb , [ ] , [ ] );  OpenFcn=sps_rtmsupport('OpenFcn',gcbh)
      mask Help: helpview(psbhelp)
      mask TypeOptions SimulationMode: Continuous | Discrete | Phasor | Discrete phasor
      mask Callback SimulationMode: powergui('SimulationType',[],[],gcb);
      mask TypeOptions UnitsV: V | kV
      mask TypeOptions UnitsW: W | kW | MW
      mask Callback CurrentSourceSwitches: powergui('SimulationType',[],[],gcb);
      mask Callback AutomaticDiscreteSolvers: powergui('SimulationType',[],[],gcb);
      mask TypeOptions SolverType: Tustin/Backward Euler (TBE) | Tustin | Backward Euler
      mask Callback SolverType: powergui('SimulationType',[],[],gcb);
      mask Callback Interpol: powergui('SimulationType',[],[],gcb);
      mask Callback ExternalGateDelay: powergui('SimulationType',[],[],gcb);
      mask Callback methode: powergui('SimulationType',[],[],gcb);
      mask TypeOptions x0status: blocks | steady | zero
      mask TypeOptions RestoreLinks: yes | warning | no
      mask Callback display: sps_rtmsupport('parametereditingmodes',gcbh) % Will be executed last in parameter callbacks to ensure mask enable consistency
      mask DialogControl SolverTab Prompt: Solver
      mask DialogControl AutoSolverNote Prompt: The Simulation type parameter is governed by Simulink. To access the Powergui solver settings, unselect auto (Automatic solver selection) solver in the Simulink solver options.
      mask DialogControl Apps Prompt: Apps
      mask DialogControl StateAnalyzer Prompt: Measurements and States Analyzer
      mask DialogControl StateAnalyzer Callback: powerStates(bdroot(gcb))
      mask DialogControl LineParameterCalculator Prompt: Line Parameter Calculator
      mask DialogControl LineParameterCalculator Callback:
      | close_system(gcb)
      | powerLineParameters
      mask DialogControl CableParameterCalculator Prompt: Cable Parameter Calculator
      mask DialogControl CableParameterCalculator Callback:
      | close_system(gcb)
      | powerCableParameters
      mask DialogControl LineDecoupler Prompt: Line Decoupler
      mask DialogControl LineDecoupler Tooltip: Click to replace selected Distributed Parameters Line blocks with Decoupling Line blocks
      mask DialogControl LineDecoupler Callback:
      | close_system(gcb);
      | DecouplingLineReplace(gcs)
      mask DialogControl LoadFlowAnalyzer Prompt: Load Flow Analyzer
      mask DialogControl LoadFlowAnalyzer Callback:
      | close_system(gcb)
      | powerLoadFlow
      mask DialogControl LoadFlowParameters Prompt: Load Flow Parameters
      mask DialogControl ImpedanceCalculator Prompt: Impedance Calculator
      mask DialogControl ImpedanceCalculator Callback:
      | close_system(gcb);
      | powerImpedance(bdroot(gcs));
      mask DialogControl FFTAnalyzer Prompt: FFT Analyzer
      mask DialogControl FFTAnalyzer Callback:
      | close_system(gcb)
      | power_fftscope(bdroot(gcb),gcb)
      mask DialogControl LinearSystemAnalyzer Prompt: Linear System Analyzer
      mask DialogControl LinearSystemAnalyzer Callback:
      | close_system(gcb)
      | power_ltiview(bdroot(gcb))
      mask DialogControl HysteresisDesigner Prompt: Hysteresis Designer
      mask DialogControl HysteresisDesigner Callback:
      | close_system(gcb)
      | powerHysteresis('hysteresis.mat')
      mask DialogControl BlockCustomizer Prompt: Block Customizer
      mask DialogControl BlockCustomizer Callback:
      | close_system(gcb);
      | power_customize;
      mask DialogControl ReportGenerator Prompt: Report Generator
      mask DialogControl ReportGenerator Callback:
      | close_system(gcb)
      | power_report(bdroot(gcb))
      mask DialogControl obsolete Prompt: ...
      mask DialogControl MachineInitialization Prompt: Machine Initialization
      mask DialogControl MachineInitialization Callback:
      | close_system(gcb)
      | powericon('machineInitTool',bdroot(gcb),gcb)
      mask DialogControl Preferences Prompt: Preferences
      mask DialogControl Solver Prompt: Solver
      mask DialogControl SolverDetails Prompt: Solver details for nonlinear elements
      mask Display: color('blue'),disp(dispMessage)
  motor_out : Outport  VectorParamsAs1DForOutWhenUnconnected=off
  wires:
  Constant1/1 -> Controlled Voltage Source1/1
  Voltage Measurement1/1 -> Vdc/1
  Permanent Magnet Synchronous Machine/1 -> motor_out/1
  Tm_Nm/1 -> Permanent Magnet Synchronous Machine/1
  gates_PWM/1 -> Universal Bridge/1
  Multimeter/1 -> Scope/1
  connections:
  Universal Bridge/LConn2 -- Permanent Magnet Synchronous Machine/LConn2
  Voltage Measurement1/LConn1 -- Controlled Voltage Source1/RConn1 -- Universal Bridge/RConn1
  Controlled Voltage Source1/LConn1 -- Voltage Measurement1/LConn2 -- Universal Bridge/RConn2
  Universal Bridge/LConn3 -- Permanent Magnet Synchronous Machine/LConn3
  Universal Bridge/LConn1 -- Permanent Magnet Synchronous Machine/LConn1
